simulink model "Sepic_Converter"  (R2016a)
settings: Solver=VariableStepAuto  StartTime=0.0  StopTime=10  RelTol=1e-3
undefined symbols (not defined in the file): Ts_Power
libraries: powerlib x13, dspstat3 x4, powerlib_meascontrol x2
settings Model: Creator=Rangga  LastModifiedBy=Rangga

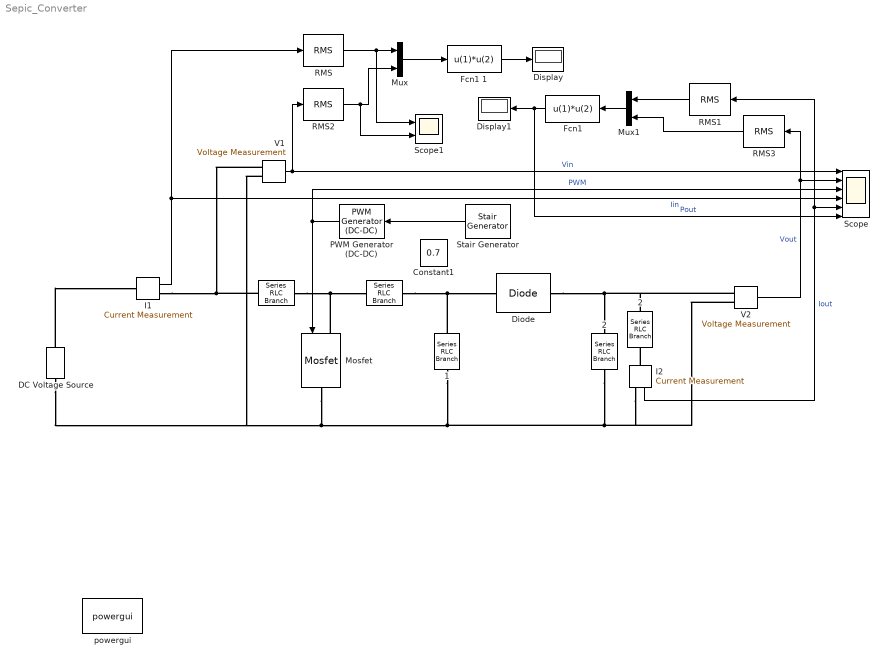
== system Sepic_Converter ==
  " " : powerlib/Elements/Series RLC Branch  LConnTagsString=__new0  RConnTagsString=__new0  BranchType=L  Resistance=2  Inductance=2.5e-3  SetiL0=off  InitialCurrent=0  Capacitance=[]  Setx0=off  InitialVoltage=0  Measurements=None
  " " : powerlib/Elements/Series RLC Branch  LConnTagsString=__new0  RConnTagsString=__new0  BranchType=C  Resistance=3000e-6  Inductance=2e-3  SetiL0=off  InitialCurrent=0  Capacitance=0.001  Setx0=off  InitialVoltage=10  Measurements=None
  " 2" : powerlib/Elements/Series RLC Branch  LConnTagsString=__new0  RConnTagsString=__new0  BranchType=C  Resistance=3000e-6  Inductance=2e-3  SetiL0=off  InitialCurrent=0  Capacitance=0.001  Setx0=off  InitialVoltage=10  Measurements=None
  " 1" : powerlib/Elements/Series RLC Branch  LConnTagsString=__new0  RConnTagsString=__new0  BranchType=L  Resistance=2  Inductance=2e-3  SetiL0=off  InitialCurrent=0  Capacitance=[]  Setx0=off  InitialVoltage=0  Measurements=None
  " 2" : powerlib/Elements/Series RLC Branch  LConnTagsString=__new0  RConnTagsString=__new0  BranchType=R  Resistance=5  Inductance=2e-3  SetiL0=off  InitialCurrent=0  Capacitance=0.01  Setx0=off  InitialVoltage=0  Measurements=None
  Constant1 : Constant  Value=0.7
  DC Voltage Source : powerlib/Electrical Sources/DC Voltage Source  Amplitude=100  Measurements=None
  Diode : powerlib/Power Electronics/Diode  Ron=0.0001  Lon=0  Vf=0.8  IC=0  UseSnubber=off  Rs=0  Cs=0  Measurements=off
  Display : Display
  Display1 : Display
  "Fcn1 " : Fcn  Expr=u(1)*u(2)
  Fcn1 1 : Fcn  Expr=u(1)*u(2)
  I1 : powerlib/Measurements/Current Measurement  Tag=PoWeRsYsTeMmEaSuReMeNt  PhasorSimulation=off  OutputType=Magnitude  PSBequivalent=0
  I2 : powerlib/Measurements/Current Measurement  Tag=PoWeRsYsTeMmEaSuReMeNt  PhasorSimulation=off  OutputType=Magnitude  PSBequivalent=0
  Mosfet : powerlib/Power Electronics/Mosfet  Ron=0.1  Lon=0  Rd=0.01  Vfd=0  IC=0  Rs=1e5  Cs=inf  Measurements=off
  Mux : Mux  Inputs=2
  Mux1 : Mux  Inputs=2
  "PWM Generator (DC-DC) " : powerlib_meascontrol/Pulse & Signal Generators/PWM Generator (DC-DC)  Fsw=60*40  Ts=0
  RMS{,1..3} (4 alike) : dspstat3/RMS  run=on  reset_popup=None  InputProcessing=Columns as channels (frame based)  directionMode=Each column  dimension=1
  Scope : Scope  NumInputPorts=6
  Scope1 : Scope  NumInputPorts=2
  Stair Generator : powerlib_meascontrol/Pulse & Signal Generators/Stair Generator  t=[0, 1, 2, 3, 4, 5, 6, 7, 8]  e=[0.1, 0.2, 0.3, 0.4, 0.5, 0.6, 0.7, 0.8, 0.9]  Ts=Ts_Power
  V1 : powerlib/Measurements/Voltage Measurement  Tag=PoWeRsYsTeMmEaSuReMeNt  PhasorSimulation=off  OutputType=Magnitude  PSBequivalent=0
  V2 : powerlib/Measurements/Voltage Measurement  Tag=PoWeRsYsTeMmEaSuReMeNt  PhasorSimulation=off  OutputType=Magnitude  PSBequivalent=0
  powergui : powerlib/powergui  Priority=1  SimulationMode=Discrete  SolverType=Tustin/Backward Euler (TBE)  SampleTime=50e-6  frequency=60  SPID=off  DisableSnubberDevices=off  DisableRonSwitches=off  DisableVfSwitches=off  SwTol=0  DisplayEquations=off  Interpol=off  ExternalGateDelay=off  methode=off  Ts=10  FunctionMessages=off  echomessages=off  HookPort=off  EnableUseOfTLC=off  x0status=blocks  frequencyindice=0  Pbase=100e6  ErrMax=1e-4  Iterations=50  UnitsV=kV  UnitsW=MW  buscounter=0  RestoreLinks=warning  ResistiveCurrentMeasurement=off  Frange=[0:2:500]  Ylog=off  Xlog=on  ShowGrid=off  save=off  variable=ZData  structure=0  ZoomFFT=off  StartTime=0.0  cycles=1  DisplayStyle=1  fundamental=60  FreqAxis=off  MaxFrequency=1000  frequencyindicesteady=1  RmsSteady=1  display=off
  wires:
  "PWM Generator (DC-DC) "/1 -> Mosfet/1, Scope/3  "PWM"
  V1/1 -> RMS2/1, Scope/1  "Vin"
  V2/1 -> RMS3/1, Scope/2  "Vout"
  I1/1 -> RMS/1, Scope/4  "Iin"
  Fcn1 1/1 -> Display/1
  I2/1 -> RMS1/1, Scope/5  "Iout"
  "Fcn1 "/1 -> Display1/1, Scope/6  "Pout"
  Mux/1 -> Fcn1 1/1
  RMS/1 -> Scope1/1, Mux/1
  RMS2/1 -> Scope1/2, Mux/2
  Mux1/1 -> "Fcn1 "/1
  RMS1/1 -> Mux1/1
  RMS3/1 -> Mux1/2
  Stair Generator/1 -> "PWM Generator (DC-DC) "/1
  connections:
  " "/RConn1 -- I1/RConn1 -- V1/LConn1
  " 1"/LConn1 -- V2/LConn2 -- I2/RConn1 -- " 2"/RConn1 -- DC Voltage Source/LConn1 -- V1/LConn2 -- Mosfet/RConn1
  " "/LConn1 -- " 1"/RConn1 -- Diode/LConn1
  Diode/RConn1 -- " 2"/LConn1 -- V2/LConn1
  " "/LConn1 -- Mosfet/LConn1 -- " "/RConn1
  I2/LConn1 -- " 2"/RConn1
  DC Voltage Source/RConn1 -- I1/LConn1
